simulink model "adaptiveCT"  (R2022a)
settings: Solver=VariableStepAuto  StartTime=0.0  StopTime=timeSpan  RelTol=1e-4
values from neighbouring files (symbols this model uses):
  B = [zeros(n);       eye(n)]    [adaptiveCT_main.m]
  K_p = 50 * eye(n)    [adaptiveCT_main.m]
  K_v = 10 * eye(n)    [adaptiveCT_main.m]
  max_tau = 100 * [1 1 1 1 1 1]    [adaptiveCT_main.m]
  P = lyap(A',Q)    [adaptiveCT_main.m]
  R = 10 * eye(n * 10)    [adaptiveCT_main.m]
undefined symbols (not defined in the file or in its folder): pi_est_0, pi_real
(part 1 of 5)
settings Model: SimulationMode=accelerator  Creator=v  LastModifiedBy=v
settings HardwareCC: ProdBitPerLong=64  ProdHWDeviceType=Intel->x86-64 (Mac OS X)

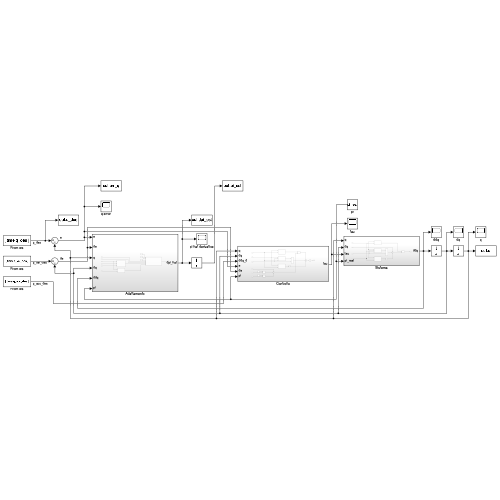
[thumbnail: Simulink's stored preview of the top-level diagram]
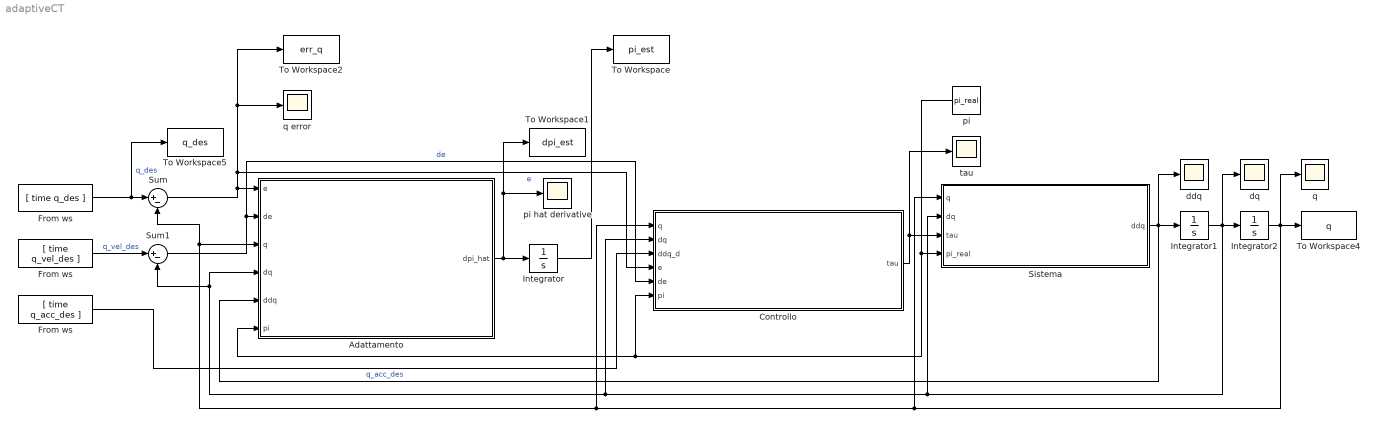
== system adaptiveCT ==
  Adattamento : Subsystem
  Controllo : Subsystem
  From ws : FromWorkspace  VariableName=[ time q_acc_des ]
  "From ws " : FromWorkspace  VariableName=[ time q_des ]
  "From ws " : FromWorkspace  VariableName=[ time q_vel_des ]
  Integrator : Integrator  InitialCondition=pi_est_0
  Integrator1 : Integrator  InitialCondition=zeros(6,1)
  Integrator2 : Integrator  InitialCondition=zeros(6,1)
  Sistema : Subsystem
  Sum : Sum  Inputs=|+-
  Sum1 : Sum  Inputs=|+-
  To Workspace : ToWorkspace  VariableName=pi_est  SaveFormat=Structure With Time  SampleTime=-1
  To Workspace1 : ToWorkspace  VariableName=dpi_est  SaveFormat=Structure With Time  SampleTime=-1
  To Workspace2 : ToWorkspace  VariableName=err_q  SaveFormat=Structure With Time  SampleTime=-1
  To Workspace4 : ToWorkspace  VariableName=q  SaveFormat=Structure With Time  SampleTime=-1
  To Workspace5 : ToWorkspace  VariableName=q_des  SaveFormat=Structure With Time  SampleTime=-1
  ddq : Scope
  dq : Scope
  pi : Constant  Value=pi_real
  pi hat derivative : Scope
  q : Scope
  q error : Scope
  tau : Scope
  wires:
  Integrator/1 -> To Workspace/1
  Adattamento/1(dpi_hat) -> Integrator/1, pi hat derivative/1, To Workspace1/1
  "From ws "/1 -> Sum/1, To Workspace5/1  "q_des"
  Integrator1/1 -> dq/1, Integrator2/1, Adattamento/4(dq), Sum1/2, Controllo/2(dq), Sistema/2(dq)
  Integrator2/1 -> To Workspace4/1, Sum/2, Adattamento/3(q), Controllo/1(q), Sistema/1(q), q/1
  Sum/1 -> Controllo/4(e), To Workspace2/1, q error/1, Adattamento/1(e)  "e"
  Sum1/1 -> Controllo/5(de), Adattamento/2(de)  "de"
  Sistema/1(ddq) -> ddq/1, Integrator1/1, Adattamento/5(ddq)
  "From ws "/1 -> Sum1/1  "q_vel_des"
  From ws/1 -> Controllo/3(ddq_d)  "q_acc_des"
  Controllo/1(tau) -> tau/1, Sistema/3(tau)
  pi/1 -> Controllo/6(pi), Adattamento/6(pi), Sistema/4(pi_real)

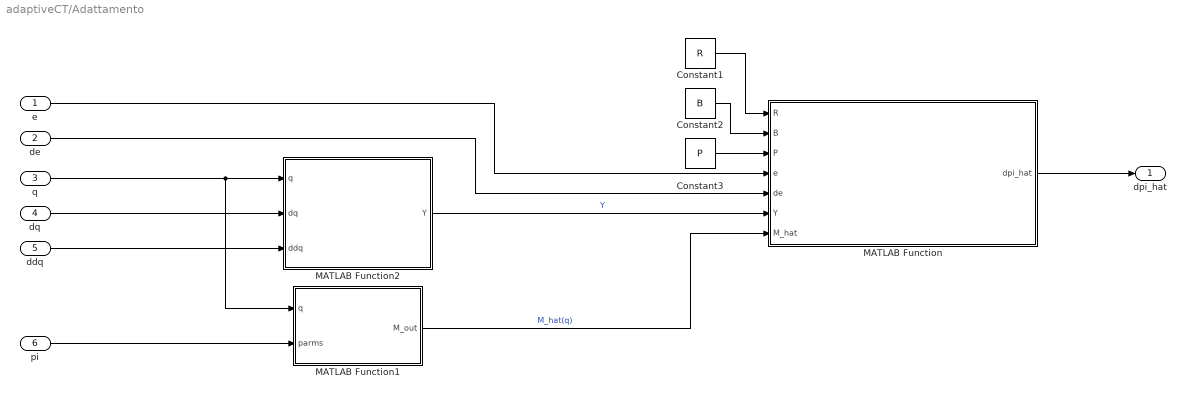
== system adaptiveCT/Adattamento ==
  e : Inport
  de : Inport  Port=2
  q : Inport  Port=3
  dq : Inport  Port=4
  ddq : Inport  Port=5
  pi : Inport  Port=6
  Constant1 : Constant  Value=R  VectorParams1D=off
  Constant2 : Constant  Value=B  VectorParams1D=off
  Constant3 : Constant  Value=P  VectorParams1D=off
  MATLAB Function : MATLAB Function  TreatAsAtomicUnit=on
  MATLAB Function1 : MATLAB Function  TreatAsAtomicUnit=on
  MATLAB Function2 : MATLAB Function  TreatAsAtomicUnit=on
  dpi_hat : Outport  VectorParamsAs1DForOutWhenUnconnected=off
  wires:
  e/1 -> MATLAB Function/4(e)
  MATLAB Function/1(dpi_hat) -> dpi_hat/1
  de/1 -> MATLAB Function/5(de)
  MATLAB Function2/1(Y) -> MATLAB Function/6(Y)  "Y"
  ddq/1 -> MATLAB Function2/3(ddq)
  dq/1 -> MATLAB Function2/2(dq)
  MATLAB Function1/1(M_out) -> MATLAB Function/7(M_hat)  "M_hat(q)"
  q/1 -> MATLAB Function1/1(q), MATLAB Function2/1(q)
  Constant1/1 -> MATLAB Function/1(R)
  Constant3/1 -> MATLAB Function/3(P)
  Constant2/1 -> MATLAB Function/2(B)
  pi/1 -> MATLAB Function1/2(parms)

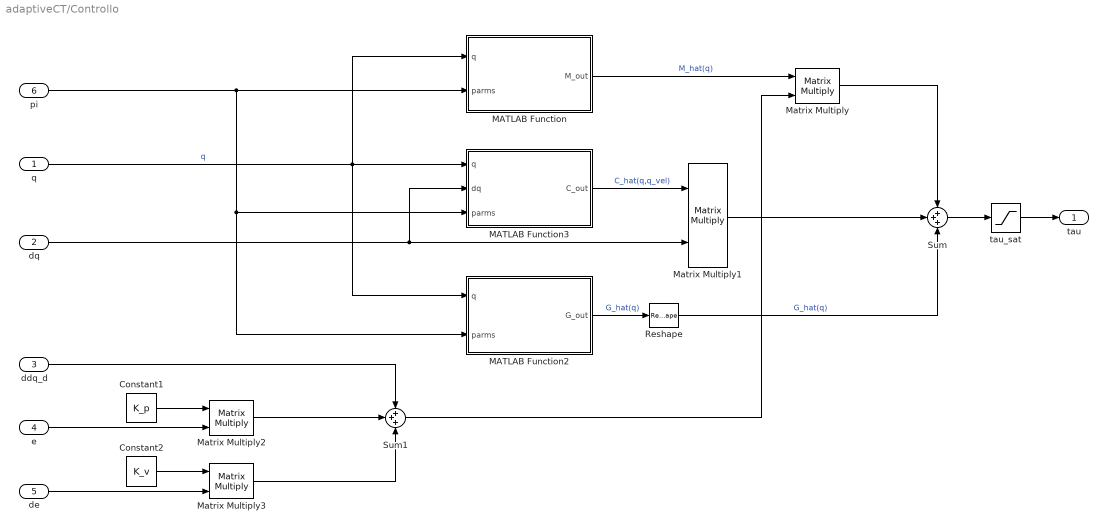
== system adaptiveCT/Controllo ==
  q : Inport
  dq : Inport  Port=2
  ddq_d : Inport  Port=3
  e : Inport  Port=4
  de : Inport  Port=5
  pi : Inport  Port=6
  Constant1 : Constant  Value=K_p  VectorParams1D=off
  Constant2 : Constant  Value=K_v  VectorParams1D=off
  MATLAB Function : MATLAB Function  TreatAsAtomicUnit=on
  MATLAB Function2 : MATLAB Function  TreatAsAtomicUnit=on
  MATLAB Function3 : MATLAB Function  TreatAsAtomicUnit=on
  Matrix Multiply{,1..3} (4 alike) : Product  Multiplication=Matrix(*)
  Reshape : Reshape
  Sum : Sum  Inputs=+++
  Sum1 : Sum  Inputs=+++
  tau_sat : Saturate  UpperLimit=max_tau  LowerLimit=-max_tau
  tau : Outport  VectorParamsAs1DForOutWhenUnconnected=off
  wires:
  Matrix Multiply/1 -> Sum/1
  Matrix Multiply1/1 -> Sum/2
  Matrix Multiply2/1 -> Sum1/2
  Matrix Multiply3/1 -> Sum1/3
  ddq_d/1 -> Sum1/1
  Sum1/1 -> Matrix Multiply/2
  q/1 -> MATLAB Function/1(q), MATLAB Function2/1(q), MATLAB Function3/1(q)  "q"
  Reshape/1 -> Sum/3  "G_hat(q)"
  MATLAB Function/1(M_out) -> Matrix Multiply/1  "M_hat(q)"
  MATLAB Function3/1(C_out) -> Matrix Multiply1/1  "C_hat(q,q_vel)"
  dq/1 -> MATLAB Function3/2(dq), Matrix Multiply1/2
  e/1 -> Matrix Multiply2/2
  Constant1/1 -> Matrix Multiply2/1
  de/1 -> Matrix Multiply3/2
  Constant2/1 -> Matrix Multiply3/1
  tau_sat/1 -> tau/1
  MATLAB Function2/1(G_out) -> Reshape/1  "G_hat(q)"
  pi/1 -> MATLAB Function2/2(parms), MATLAB Function3/3(parms), MATLAB Function/2(parms)
  Sum/1 -> tau_sat/1

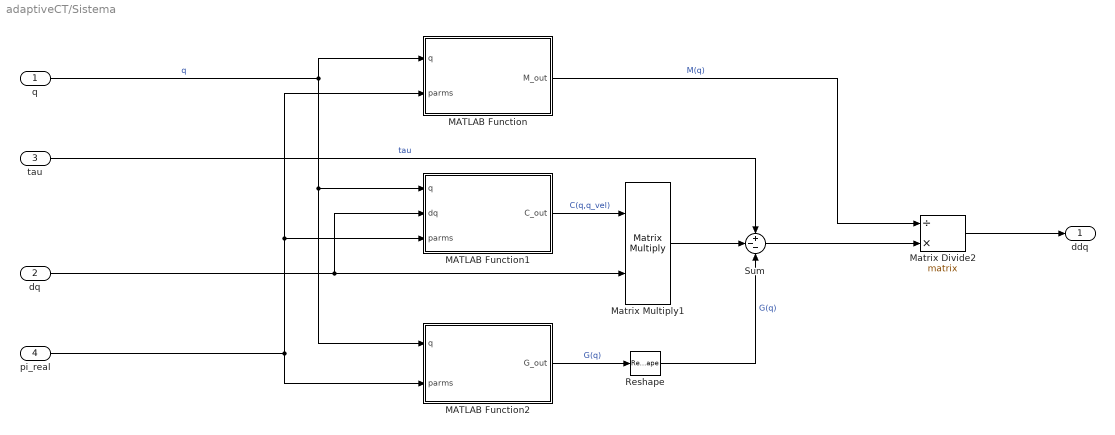
== system adaptiveCT/Sistema ==
  q : Inport
  dq : Inport  Port=2
  tau : Inport  Port=3
  pi_real : Inport  Port=4
  MATLAB Function : MATLAB Function  TreatAsAtomicUnit=on
  MATLAB Function1 : MATLAB Function  TreatAsAtomicUnit=on
  MATLAB Function2 : MATLAB Function  TreatAsAtomicUnit=on
  Matrix Divide2 : Product  Inputs=/*  Multiplication=Matrix(*)
  Matrix Multiply1 : Product  Multiplication=Matrix(*)
  Reshape : Reshape
  Sum : Sum  Inputs=+--
  ddq : Outport  VectorParamsAs1DForOutWhenUnconnected=off
  wires:
  tau/1 -> Sum/1  "tau"
  Matrix Multiply1/1 -> Sum/2
  Sum/1 -> Matrix Divide2/2
  dq/1 -> MATLAB Function1/2(dq), Matrix Multiply1/2
  Matrix Divide2/1 -> ddq/1
  q/1 -> MATLAB Function2/1(q), MATLAB Function1/1(q), MATLAB Function/1(q)  "q"
  MATLAB Function1/1(C_out) -> Matrix Multiply1/1  "C(q,q_vel)"
  Reshape/1 -> Sum/3  "G(q)"
  MATLAB Function/1(M_out) -> Matrix Divide2/1  "M(q)"
  pi_real/1 -> MATLAB Function/2(parms), MATLAB Function1/3(parms), MATLAB Function2/2(parms)
  MATLAB Function2/1(G_out) -> Reshape/1  "G(q)"
